simulink model "control"  (R2022b)
settings: Solver=VariableStepAuto  StartTime=0.0  StopTime=10.0  RelTol=1e-3
values from neighbouring files (symbols this model uses):
  q0 = [-0.9273 -1.287 0.7 2.2143]    [generated_traj.mat]
  Tc = 0.001    [generated_traj.mat]
undefined symbols (not defined in the file or in its folder): DiscIntNeverNeededParam
settings Model: Creator=giuseppeloianno  LastModifiedBy=shubham

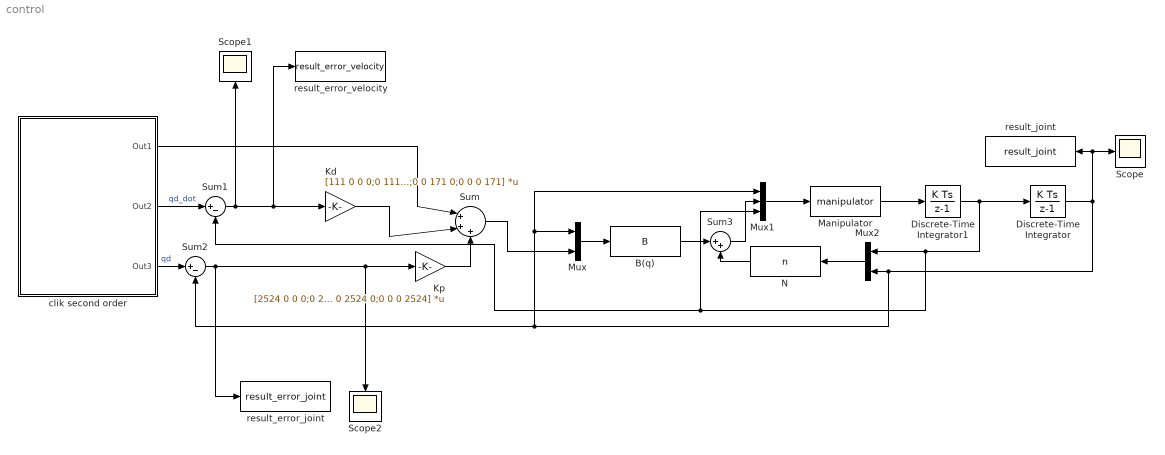
== system control ==
  B(q) : MATLABFcn  MATLABFcn=B  OutputDimensions=4
  Discrete-Time Integrator : DiscreteIntegrator  InitialCondition=q0  SampleTime=Tc  LimitOutput=on  UpperSaturationLimit=[inf;inf;inf;inf]  LowerSaturationLimit=[-inf;-inf;-inf;-inf]  ICPrevOutput=DiscIntNeverNeededParam  ICPrevScaledInput=DiscIntNeverNeededParam
  Discrete-Time Integrator1 : DiscreteIntegrator  InitialCondition=q0  SampleTime=0.001  ICPrevOutput=DiscIntNeverNeededParam  ICPrevScaledInput=DiscIntNeverNeededParam
  Kd : Gain  Gain=[111 0 0 0;0 111 0 0;0 0 171 0;0 0 0 171]  Multiplication=Matrix(K*u)
  Kp : Gain  Gain=[2524 0 0 0;0 2524 0 0;0 0 2524 0;0 0 0 2524]  Multiplication=Matrix(K*u)
  Manipulator : MATLABFcn  MATLABFcn=manipulator  OutputDimensions=4
  Mux : Mux  Inputs=2
  Mux1 : Mux  Inputs=3
  Mux2 : Mux  Inputs=2
  N : MATLABFcn  MATLABFcn=n  OutputDimensions=4
  Scope : Scope
  Scope1 : Scope
  Scope2 : Scope
  Sum : Sum  Inputs=|+++
  Sum1 : Sum  Inputs=|+-
  Sum2 : Sum  Inputs=|+-
  Sum3 : Sum  Inputs=|++
  clik second order : Subsystem
  result_error_joint : ToWorkspace  VariableName=result_error_joint  SampleTime=-1
  result_error_velocity : ToWorkspace  VariableName=result_error_velocity  SampleTime=-1
  result_joint : ToWorkspace  VariableName=result_joint  SampleTime=-1
  wires:
  Mux1/1 -> Manipulator/1
  B(q)/1 -> Sum3/1
  Kp/1 -> Sum/3
  clik second order/2(Out2) -> Sum1/1  "qd_dot"
  Sum/1 -> Mux/2
  Mux/1 -> B(q)/1
  Sum2/1 -> Scope2/1, Kp/1, result_error_joint/1
  Mux2/1 -> N/1
  Sum1/1 -> Kd/1, result_error_velocity/1, Scope1/1
  Kd/1 -> Sum/2
  clik second order/1(Out1) -> Sum/1
  Discrete-Time Integrator/1 -> Mux2/2, Mux1/1, Mux/1, Sum2/2, Scope/1, result_joint/1
  Sum3/1 -> Mux1/2
  N/1 -> Sum3/2
  clik second order/3(Out3) -> Sum2/1  "qd"
  Discrete-Time Integrator1/1 -> Mux2/1, Mux1/3, Sum1/2, Discrete-Time Integrator/1
  Manipulator/1 -> Discrete-Time Integrator1/1

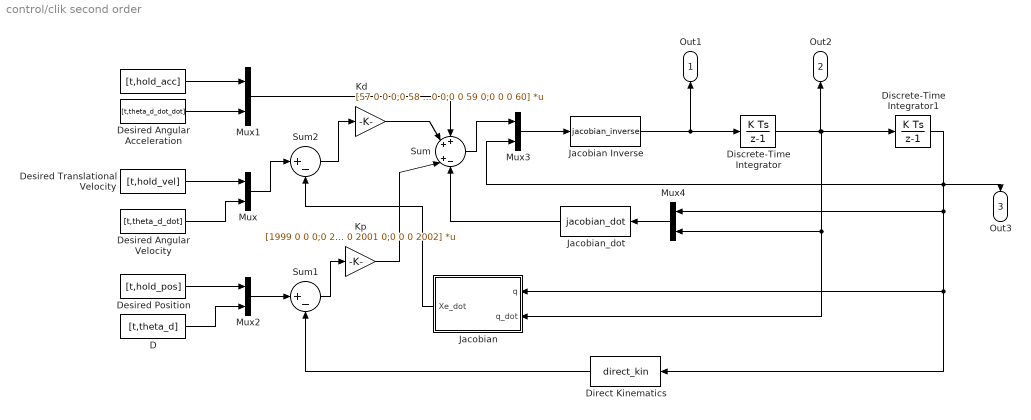
== system control/clik second order ==
  " " : FromWorkspace  VariableName=[t,hold_acc]  SampleTime=0.001
  D : FromWorkspace  VariableName=[t,theta_d]  SampleTime=0.001
  Desired Angular Acceleration : FromWorkspace  VariableName=[t,theta_d_dot_dot]  SampleTime=0.001
  Desired Angular Velocity : FromWorkspace  VariableName=[t,theta_d_dot]  SampleTime=0.001
  Desired Position : FromWorkspace  VariableName=[t,hold_pos]  SampleTime=0.001
  Desired Translational Velocity : FromWorkspace  VariableName=[t,hold_vel]  SampleTime=0.001
  Direct Kinematics : MATLABFcn  MATLABFcn=direct_kin  OutputDimensions=4
  Discrete-Time Integrator : DiscreteIntegrator  InitialCondition=q0  SampleTime=Tc  ICPrevOutput=DiscIntNeverNeededParam  ICPrevScaledInput=DiscIntNeverNeededParam
  Discrete-Time Integrator1 : DiscreteIntegrator  InitialCondition=q0  SampleTime=Tc  ICPrevOutput=DiscIntNeverNeededParam  ICPrevScaledInput=DiscIntNeverNeededParam
  "Jacobian " : MATLAB Function  TreatAsAtomicUnit=on
  Jacobian Inverse : MATLABFcn  MATLABFcn=jacobian_inverse  OutputDimensions=4
  Jacobian_dot : MATLABFcn  MATLABFcn=jacobian_dot  OutputDimensions=4
  Kd : Gain  Gain=[57 0 0 0;0 58 0 0;0 0 59 0;0 0 0 60]  Multiplication=Matrix(K*u)
  Kp : Gain  Gain=[1999 0 0 0;0 2000 0 0;0 0 2001 0;0 0 0 2002]  Multiplication=Matrix(K*u)
  Mux{,1..4} (5 alike) : Mux  Inputs=2
  Sum : Sum  Inputs=++|+-
  Sum1 : Sum  Inputs=|+-
  Sum2 : Sum  Inputs=|+-
  Out1 : Outport
  Out2 : Outport  Port=2
  Out3 : Outport  Port=3
  wires:
  Sum1/1 -> Kp/1
  Desired Angular Acceleration/1 -> Mux1/2
  Sum2/1 -> Kd/1
  Desired Angular Velocity/1 -> Mux/2
  Jacobian_dot/1 -> Sum/4
  Mux/1 -> Sum2/1
  Mux2/1 -> Sum1/1
  D/1 -> Mux2/2
  Discrete-Time Integrator1/1 -> Mux4/1, "Jacobian "/1(q), Direct Kinematics/1, Out3/1, Mux3/2
  Sum/1 -> Mux3/1
  Mux3/1 -> Jacobian Inverse/1
  Kp/1 -> Sum/3
  Mux4/1 -> Jacobian_dot/1
  " "/1 -> Mux1/1
  Discrete-Time Integrator/1 -> Discrete-Time Integrator1/1, "Jacobian "/2(q_dot), Mux4/2, Out2/1
  Mux1/1 -> Sum/1
  Desired Translational Velocity/1 -> Mux/1
  Kd/1 -> Sum/2
  Desired Position/1 -> Mux2/1
  Direct Kinematics/1 -> Sum1/2
  "Jacobian "/1(Xe_dot) -> Sum2/2
  Jacobian Inverse/1 -> Discrete-Time Integrator/1, Out1/1

== matlab function control/clik second order/Jacobian  ==
  data: q input; Xe_dot output; q_dot input
function Xe_dot= fcn(q,q_dot)
    % given angles
    theta1=q(1);
    theta2=q(2);
    % given inputs
    a1=0.5;
    a2=0.5;
    
    jacobian_mat=[- a2*sin(theta1 + theta2) - a1*sin(theta1), -a2*sin(theta1 + theta2), 0, 0; 
        a2*cos(theta1 + theta2) + a1*cos(theta1), a2*cos(theta1 + theta2), 0,0; 
        0, 0, -1, 0;
        1, 1, 0, 1];
    
    Xe_dot=jacobian_mat*q_dot;

end
